simulink model "Gradient_Identification"  (R2015b)
settings: Solver=VariableStepAuto  StartTime=0.0  StopTime=10000  FixedStep=1/100  RelTol=1e-3
values from neighbouring files (symbols this model uses):
  cell_A123 =     [cells.mat]
  cell_sanyo =     [cells.mat]
libraries: simulink x6, dspfdesign x2
settings Model: Creator=eprakE  LastModifiedBy=eprakE
settings DebuggingCC: InheritedTsInSrcMsg=none

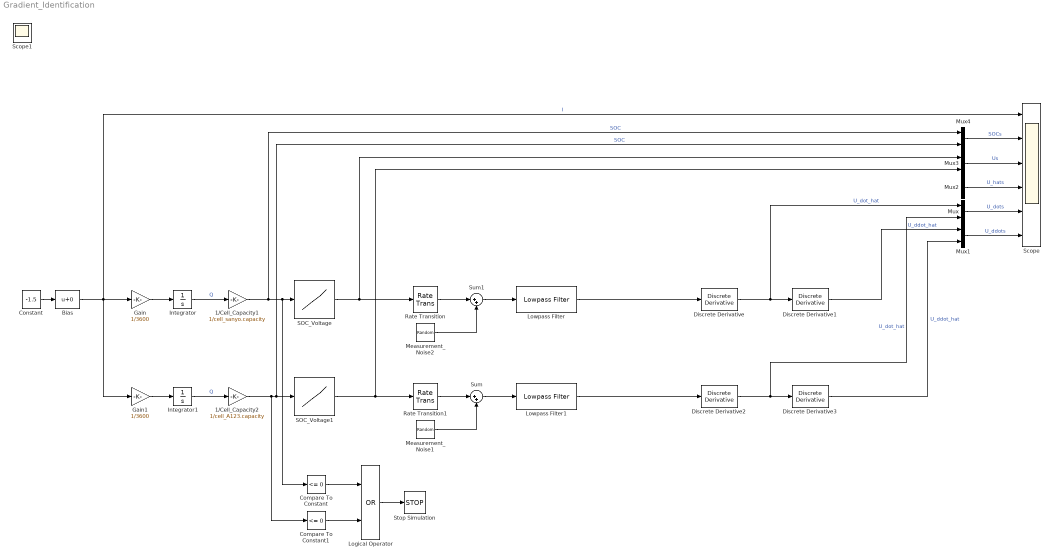
== system Gradient_Identification ==
  1/Cell_Capacity1 : Gain  Gain=1/cell_sanyo.capacity
  1/Cell_Capacity2 : Gain  Gain=1/cell_A123.capacity
  Bias : Bias
  Compare To Constant : simulink/Logic and Bit Operations/Compare To Constant  relop=<=  const=0  OutDataTypeStr=boolean
  Compare To Constant1 : simulink/Logic and Bit Operations/Compare To Constant  relop=<=  const=0  OutDataTypeStr=boolean
  Constant : Constant  Value=-1.5
  Discrete Derivative{,1..3} (4 alike) : simulink/Discrete/Discrete Derivative  gainval=1.0  ICPrevScaledInput=0.0  InputProcessing=Inherited  OutMin=[]  OutMax=[]  OutDataType=fixdt(1, 16)  OutScaling=2^-10  DoSatur=off
  Gain : Gain  Gain=1/3600
  Gain1 : Gain  Gain=1/3600
  Integrator : Integrator  InitialCondition=2
  Integrator1 : Integrator  InitialCondition=1
  Logical Operator : Logic  Operator=OR  AllPortsSameDT=off  OutDataTypeStr=boolean
  Lowpass Filter : dspfdesign/Lowpass Filter  FilterType=IIR  DesignForMinimumOrder=on  FilterOrder=50  PassbandFrequency=10e-3  StopbandFrequency=1  PassbandRipple=0.1  StopbandAttenuation=60  InheritSampleRate=off  SampleRate=32e3  roundingMode=Floor  coeffsDataTypeStr=fixdt(1,16)  SimulateUsing=Interpreted execution
  Lowpass Filter1 : dspfdesign/Lowpass Filter  FilterType=IIR  DesignForMinimumOrder=on  FilterOrder=50  PassbandFrequency=10e-3  StopbandFrequency=100e-3  PassbandRipple=0.1  StopbandAttenuation=60  InheritSampleRate=off  SampleRate=100  roundingMode=Floor  coeffsDataTypeStr=fixdt(1,16)  SimulateUsing=Interpreted execution
  Measurement_Noise1 : RandomNumber  Variance=1e-6  Seed=100  SampleTime=1/32e3
  Measurement_Noise2 : RandomNumber  Variance=1e-6  SampleTime=1/32e3
  Mux{,1..4} (5 alike) : Mux  Inputs=2
  Rate Transition : RateTransition  OutPortSampleTime=1/32e3
  Rate Transition1 : RateTransition  OutPortSampleTime=1/32e3
  SOC_Voltage : Lookup_n-D  NumberOfTableDimensions=1  BreakpointsForDimension1=cell_sanyo.soc  BeginIndexSearchUsingPreviousIndexResult=on  Table=cell_sanyo.voltage  InternalRulePriority=Speed  RndMeth=Simplest  InputSameDT=on
  SOC_Voltage1 : Lookup_n-D  NumberOfTableDimensions=1  BreakpointsForDimension1=cell_A123.soc  BeginIndexSearchUsingPreviousIndexResult=on  Table=cell_A123.voltage  InternalRulePriority=Speed  RndMeth=Simplest  InputSameDT=on
  Scope : Scope  NumInputPorts=6
  Stop Simulation : Stop
  Sum : Sum  Inputs=|++
  Sum1 : Sum  Inputs=|++
  Scope1 : Scope
  wires:
  Integrator/1 -> 1/Cell_Capacity1/1  "Q"
  1/Cell_Capacity1/1 -> Compare To Constant/1, SOC_Voltage/1, Mux4/1  "SOC"
  Constant/1 -> Bias/1
  SOC_Voltage/1 -> Rate Transition/1, Mux3/1
  Bias/1 -> Gain/1, Gain1/1, Scope/1  "I"
  Discrete Derivative/1 -> Mux/1, Discrete Derivative1/1  "U_dot_hat"
  Discrete Derivative1/1 -> Mux1/1  "U_ddot_hat"
  Lowpass Filter/1 -> Discrete Derivative/1
  Discrete Derivative2/1 -> Mux/2, Discrete Derivative3/1  "U_dot_hat"
  Discrete Derivative3/1 -> Mux1/2  "U_ddot_hat"
  Lowpass Filter1/1 -> Discrete Derivative2/1
  Mux/1 -> Scope/5  "U_dots"
  Mux1/1 -> Scope/6  "U_ddots"
  Integrator1/1 -> 1/Cell_Capacity2/1  "Q"
  1/Cell_Capacity2/1 -> Compare To Constant1/1, Mux4/2, SOC_Voltage1/1  "SOC"
  Logical Operator/1 -> Stop Simulation/1
  Compare To Constant/1 -> Logical Operator/1
  Compare To Constant1/1 -> Logical Operator/2
  Mux2/1 -> Scope/4  "U_hats"
  SOC_Voltage1/1 -> Rate Transition1/1, Mux3/2
  Mux3/1 -> Scope/3  "Us"
  Mux4/1 -> Scope/2  "SOCs"
  Rate Transition/1 -> Sum1/1
  Rate Transition1/1 -> Sum/1
  Sum1/1 -> Lowpass Filter/1
  Measurement_Noise2/1 -> Sum1/2
  Measurement_Noise1/1 -> Sum/2
  Gain/1 -> Integrator/1
  Gain1/1 -> Integrator1/1
  Sum/1 -> Lowpass Filter1/1
